simulink model "Youbot2017_2016a"  (R2022a)
settings: Solver=FixedStepAuto  StartTime=0.0  StopTime=inf  RelTol=1e-3  EnableMultiTasking=on
libraries: simulink x25, simulink_extras x7, embedlinuxNetworklib x3, dspnetwork x2
settings Model: SimulationMode=external  ExtModeTrigDuration=100  Creator=svra0001  LastModifiedBy=maximilian
settings SolverCC: AlgebraicLoopSolver=TrustRegion  PositivePriorityOrder=on  AutoInsertRateTranBlk=on
settings DataIOCC: LimitDataPoints=on  SaveFormat=Array  SignalLoggingSaveFormat=ModelDataLogs  ReturnWorkspaceOutputs=off
settings OptimizationCC: UseFloatMulNetSlope=on  EfficientFloat2IntCast=on  LifeSpan=inf  MaxStackSize=64
settings DebuggingCC: UnderspecifiedInitializationDetection=Classic  MergeDetectMultiDrivingBlocksExec=none  MultiTaskDSMMsg=warning  MultiTaskCondExecSysMsg=none  ParameterTunabilityLossMsg=error  UnconnectedInputMsg=warning  UnconnectedOutputMsg=warning  UnconnectedLineMsg=warning  AllowSymbolicDim=off  StateNameClashWarn=warning  SFUnexpectedBacktrackingDiag=warning  SFNoUnconditionalDefaultTransitionDiag=warning  SFMachineParentedDataDiag=warning  ArithmeticOperatorsInVariantConditions=warning
settings HardwareCC: ProdBitPerPointer=32  ProdBitPerSizeT=32  ProdBitPerPtrDiffT=32  ProdLargestAtomicInteger=Long  ProdLargestAtomicFloat=Double  ProdWordSize=32  ProdHWDeviceType=ARM Compatible->ARM Cortex  UseEmbeddedCoderFeatures=off  UseSimulinkCoderFeatures=off
settings ModelReferenceCC: PropagateSignalLabelsOutOfModel=off
settings SFSimCC: SimUseLocalCustomCode=off  MATLABDynamicMemAlloc=off  CustomCodeGlobalsAsFunctionIO=on  DefaultCustomCodeDeterministicFunctions=All  SimTargetLang=C++
settings RTWCC: SystemTargetFile=ert.tlc  HardwareBoard=Raspberry Pi  TLCOptions="-aInlineSetEventsForThisBaseRateFcn=TLC_FALSE -aSuppressMultiTaskScheduler=TLC_FALSE  -aRateBasedStepFcn=0"  PackageName=code.zip  TemplateMakefile=ert_default_tmf  RTWVerbose=off  RTWUseLocalCustomCode=off  Toolchain=GNU GCC Embedded Linux  DLArmComputeVersion=19.05
settings CodeAppCC: ForceParamTrailComments=on  OperatorAnnotations=on  MangleLength=10  StateflowObjectComments=on  MATLABSourceComments=on
settings ERTTargetCC: MultiwordLength=2048  ERTCustomFileBanners=off  SupportContinuousTime=on  SupportNonInlinedSFcns=on  RemoveResetFunc=off  SupportVariableSizeSignals=on  ModelStepFunctionPrototypeControlCompliant=off  ExtMode=on  ExtModeMexArgs='192.168.0.4' 1 17725  ERTSrcFileBannerTemplate=codertarget_code_template.cgt  ERTHdrFileBannerTemplate=codertarget_code_template.cgt  ERTDataSrcFileTemplate=codertarget_code_template.cgt  ERTDataHdrFileTemplate=codertarget_code_template.cgt
settings ConfigComp: CovMetricSettings=dw  CovSaveCumulativeToWorkspaceVar=on  CovSaveSingleToWorkspaceVar=on  CovExternalEMLEnable=off

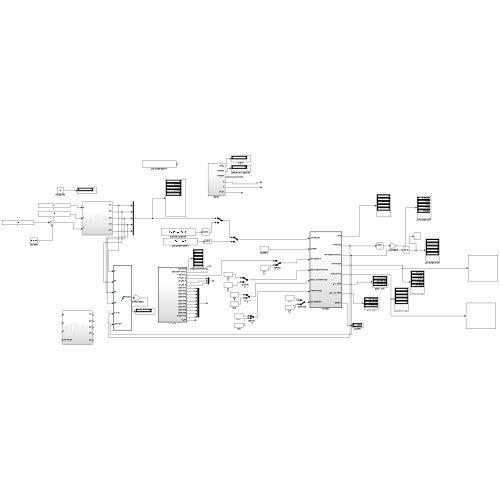
[thumbnail: Simulink's stored preview of the top-level diagram]
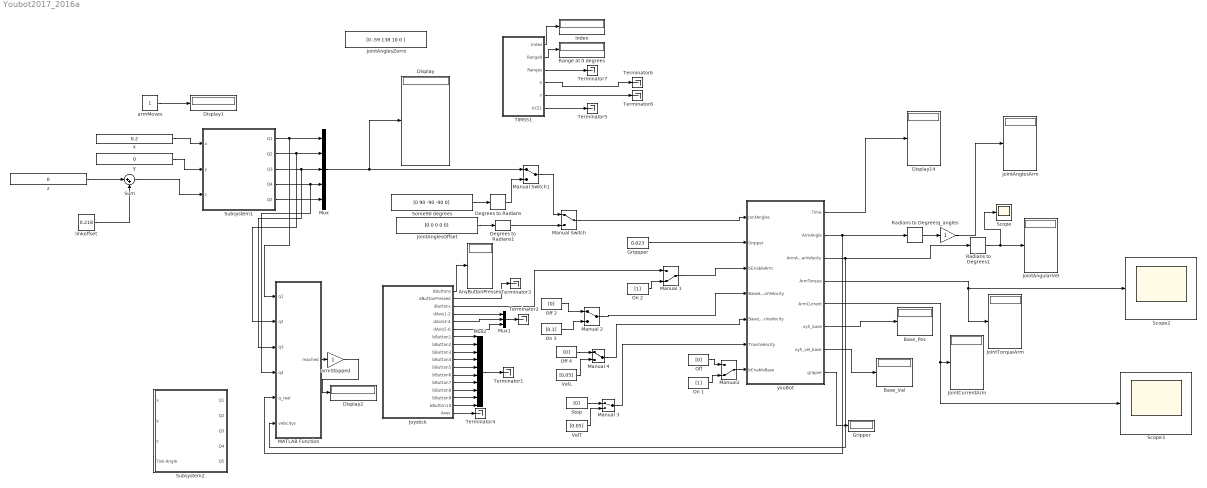
== system Youbot2017_2016a ==
  AnyButtonPressed : Display
  Base_Pos : Display
  Base_Val : Display
  Degrees to Radians : simulink_extras/Transformations/Degrees to Radians
  Degrees to Radians1 : simulink_extras/Transformations/Degrees to Radians
  Display{,1..2,14} (4 alike) : Display
  "Gripper " : Display
  Grippper : Constant  Value=0.023
  Index : Display
  JointAnglesArm : Display
  "JointAnglesOffset " : Constant  Value=[0 0 0 0 0]
  "JointAnglesZerro " : Constant  Value=[0 -59 138 10 0 ]
  JointAngularVel : Display
  JointCurrentArm : Display
  "JointTorqueArm " : Display
  "Joystick " : Subsystem  TreatAsAtomicUnit=on
      settings: RTWFcnNameOpts=Use subsystem name  RTWFileNameOpts=Use function name
  MATLAB Function : MATLAB Function  TreatAsAtomicUnit=on
  Manual 1 : ManualSwitch  CurrentSetting=0
  Manual 2 : ManualSwitch
  Manual 3 : ManualSwitch
  Manual 4 : ManualSwitch
  Manual Switch : ManualSwitch
  Manual Switch1 : ManualSwitch
  "Manual2 " : ManualSwitch  CurrentSetting=0
  Mux : Mux  Inputs=5
  Mux1 : Mux  Inputs=[2 2 2]
  Mux2 : Mux  Inputs=[1 1 1 1 1 1 1 1 1 1]
  "Off " : Constant  Value=[0]
  Off 2 : Constant  Value=[0]
  Off 4 : Constant  Value=[0]
  On 1 : Constant  Value=[1]
  On 2 : Constant  Value=[1]
  On 3 : Constant  Value=[0.1]
  Radians to Degrees : simulink_extras/Transformations/Radians to Degrees
  Radians to Degrees1 : simulink_extras/Transformations/Radians to Degrees
  "Range at 0 degrees " : Display
  Scope : Scope
  Scope2 : Scope
  Scope3 : Scope
  Some90 degrees : Constant  Value=[0 90 -90 -90 0]
  "Stop " : Constant  Value=[0]
  Subsystem1 : Subsystem
  Subsystem2 : Subsystem
  Sum : Sum  Inputs=|++
  TIM551 : Subsystem
  Terminator{1..8} (8 alike) : Terminator
  VelL : Constant  Value=[0.05]
  "VelT " : Constant  Value=[0.05]
  "armMoves " : Constant
  armStopped : Gain
  linkoffset : Constant  Value=0.218
  q_angles : Gain
  x : Constant  Value=0.2
  y : Constant  Value=0
  "youBot " : Subsystem  TreatAsAtomicUnit=on
  z : Constant  Value=0
  wires:
  Radians to Degrees/1 -> q_angles/1
  Radians to Degrees1/1 -> Scope/1, JointAngularVel/1
  "youBot "/1(Time) -> Display14/1
  "youBot "/2(ArmAngle) -> Radians to Degrees/1, MATLAB Function/5(q_real)
  "youBot "/3(ArmAngularVelocity) -> MATLAB Function/6(velocitys), Radians to Degrees1/1
  Some90 degrees/1 -> Degrees to Radians/1
  "JointAnglesOffset "/1 -> Degrees to Radians1/1
  Degrees to Radians1/1 -> Manual Switch/2
  Manual Switch/1 -> "youBot "/1(JontAngles)
  "youBot "/5(ArmCurrent) -> Scope3/1, JointCurrentArm/1
  "youBot "/4(ArmTorque) -> "JointTorqueArm "/1, Scope2/1
  "youBot "/8(gripper) -> "Gripper "/1
  "Manual2 "/1 -> "youBot "/7(bEnableBase)
  "Off "/1 -> "Manual2 "/1
  On 1/1 -> "Manual2 "/2
  On 2/1 -> Manual 1/2
  Manual 1/1 -> "youBot "/3(bEnableArm)
  Off 2/1 -> Manual 2/1
  On 3/1 -> Manual 2/2
  Manual 2/1 -> "youBot "/4("BaseAngularVelocity ")
  "Stop "/1 -> Manual 3/1
  "VelT "/1 -> Manual 3/2
  Manual 3/1 -> "youBot "/6(TransVelocity)
  Mux/1 -> Manual Switch1/1, Display/1
  Degrees to Radians/1 -> Manual Switch1/2
  Manual Switch1/1 -> Manual Switch/1
  Grippper/1 -> "youBot "/2(Gripper)
  Off 4/1 -> Manual 4/1
  VelL/1 -> Manual 4/2
  Manual 4/1 -> "youBot "/5(BaseLinearVeolocity)
  "youBot "/6(xyh_base) -> Base_Pos/1
  "youBot "/7(xyh_vel_base) -> Base_Val/1
  "Joystick "/1(bButtons) -> AnyButtonPressed/1
  "Joystick "/17(Axes) -> Terminator4/1
  "Joystick "/12(bButton6) -> Mux2/6
  "Joystick "/2("dButtonPressed ") -> Terminator3/1
  "Joystick "/7(bButton1) -> Mux2/1
  "Joystick "/8(bButton2) -> Mux2/2
  "Joystick "/9(bButton3) -> Mux2/3
  "Joystick "/10(bButton4) -> Mux2/4
  "Joystick "/11(bButton5) -> Mux2/5
  "Joystick "/13(bButton7) -> Mux2/7
  "Joystick "/14(bButton8) -> Mux2/8
  "Joystick "/15(bButton9) -> Mux2/9
  "Joystick "/16(bButton10) -> Mux2/10
  Mux2/1 -> Terminator1/1
  "Joystick "/4(dAxis1-2) -> Mux1/1
  "Joystick "/5(dAxis3-4) -> Mux1/2
  "Joystick "/6(dAxis5-6) -> Mux1/3
  Mux1/1 -> Terminator2/1
  "Joystick "/3("iButtons ") -> Manual 1/1
  TIM551/1(Index) -> Index/1
  TIM551/2(Range0) -> "Range at 0 degrees "/1
  TIM551/6(XYZ1) -> Terminator5/1
  TIM551/3(Ranges) -> Terminator7/1
  TIM551/5(Y) -> Terminator8/1
  TIM551/4(X) -> Terminator6/1
  Subsystem1/1(Q1) -> MATLAB Function/1(q1), Mux/1
  Subsystem1/3(Q3) -> MATLAB Function/3(q3), Mux/3
  Subsystem1/2(Q2) -> MATLAB Function/2(q2), Mux/2
  Subsystem1/4(Q4) -> MATLAB Function/4(q4), Mux/4
  Subsystem1/5(Q5) -> Mux/5
  "armMoves "/1 -> Display1/1
  MATLAB Function/1(reached) -> armStopped/1
  armStopped/1 -> Display2/1
  q_angles/1 -> JointAnglesArm/1
  x/1 -> Subsystem1/1(x)
  y/1 -> Subsystem1/2(y)
  z/1 -> Sum/1
  Sum/1 -> Subsystem1/3(z)
  linkoffset/1 -> Sum/2

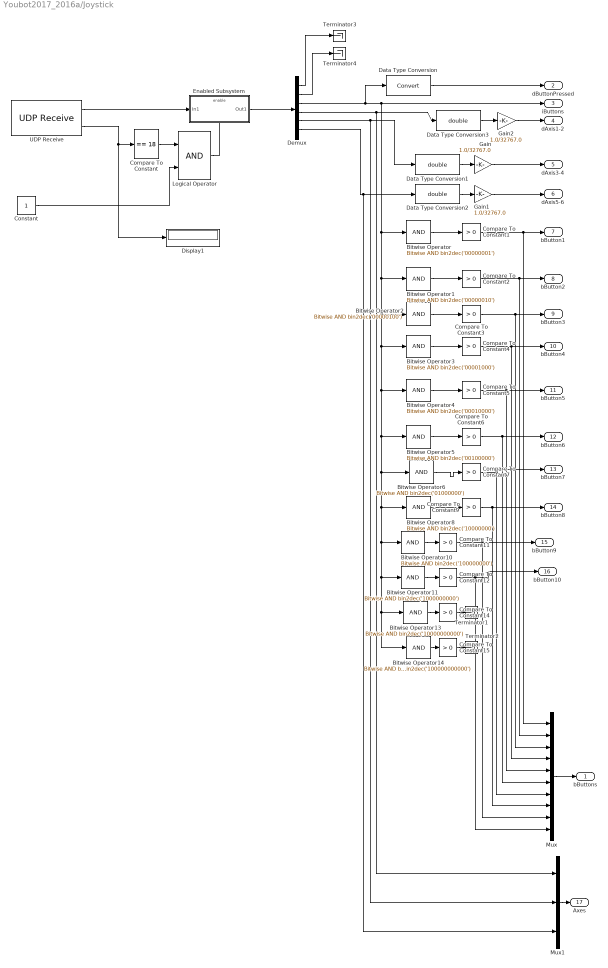
== system Youbot2017_2016a/Joystick  ==
  Bitwise Operator : simulink/Logic and Bit Operations/Bitwise Operator  logicop=AND  UseBitMask=on  BitMask=bin2dec('00000001')  BitMaskRealWorld=Stored Integer
  Bitwise Operator1 : simulink/Logic and Bit Operations/Bitwise Operator  logicop=AND  UseBitMask=on  BitMask=bin2dec('00000010')  BitMaskRealWorld=Stored Integer
  Bitwise Operator10 : simulink/Logic and Bit Operations/Bitwise Operator  logicop=AND  UseBitMask=on  BitMask=bin2dec('100000000')  BitMaskRealWorld=Stored Integer
  Bitwise Operator11 : simulink/Logic and Bit Operations/Bitwise Operator  logicop=AND  UseBitMask=on  BitMask=bin2dec('1000000000')  BitMaskRealWorld=Stored Integer
  Bitwise Operator13 : simulink/Logic and Bit Operations/Bitwise Operator  logicop=AND  UseBitMask=on  BitMask=bin2dec('10000000000')  BitMaskRealWorld=Stored Integer
  Bitwise Operator14 : simulink/Logic and Bit Operations/Bitwise Operator  logicop=AND  UseBitMask=on  BitMask=bin2dec('100000000000')  BitMaskRealWorld=Stored Integer
  Bitwise Operator2 : simulink/Logic and Bit Operations/Bitwise Operator  logicop=AND  UseBitMask=on  BitMask=bin2dec('00000100')  BitMaskRealWorld=Stored Integer
  Bitwise Operator3 : simulink/Logic and Bit Operations/Bitwise Operator  logicop=AND  UseBitMask=on  BitMask=bin2dec('00001000')  BitMaskRealWorld=Stored Integer
  Bitwise Operator4 : simulink/Logic and Bit Operations/Bitwise Operator  logicop=AND  UseBitMask=on  BitMask=bin2dec('00010000')  BitMaskRealWorld=Stored Integer
  Bitwise Operator5 : simulink/Logic and Bit Operations/Bitwise Operator  logicop=AND  UseBitMask=on  BitMask=bin2dec('00100000')  BitMaskRealWorld=Stored Integer
  Bitwise Operator6 : simulink/Logic and Bit Operations/Bitwise Operator  logicop=AND  UseBitMask=on  BitMask=bin2dec('01000000')  BitMaskRealWorld=Stored Integer
  Bitwise Operator8 : simulink/Logic and Bit Operations/Bitwise Operator  logicop=AND  UseBitMask=on  BitMask=bin2dec('10000000')  BitMaskRealWorld=Stored Integer
  Compare To Constant : simulink/Logic and Bit Operations/Compare To Constant  relop===  const=18  OutDataTypeStr=boolean
  Compare To Constant{1..7,9,11..12,14..15} (12 alike) : simulink/Logic and Bit Operations/Compare To Constant  relop=>  const=0  OutDataTypeStr=boolean
  Constant : Constant
  Data Type Conversion : DataTypeConversion  SaturateOnIntegerOverflow=off  RndMeth=Floor
  Data Type Conversion1 : DataTypeConversion  OutDataTypeStr=double  SaturateOnIntegerOverflow=off  RndMeth=Floor
  Data Type Conversion2 : DataTypeConversion  OutDataTypeStr=double  SaturateOnIntegerOverflow=off  RndMeth=Floor
  Data Type Conversion3 : DataTypeConversion  OutDataTypeStr=double  SaturateOnIntegerOverflow=off  RndMeth=Floor
  Demux : Demux  Outputs=[1 1 1 2 2 2]
  Display1 : Display
  Enabled Subsystem : Subsystem  TreatAsAtomicUnit=on
  Gain : Gain  Gain=1.0/32767.0
  Gain1 : Gain  Gain=1.0/32767.0
  Gain2 : Gain  Gain=1.0/32767.0
  Logical Operator : Logic  AllPortsSameDT=off  OutDataTypeStr=boolean
  Mux : Mux  Inputs=10
  Mux1 : Mux  Inputs=3
  Terminator{1..4} (4 alike) : Terminator
  UDP Receive : embedlinuxNetworklib/UDP Receive  localURL='0.0.0.0'  localPort=25060  remoteURL='0.0.0.0'  remotePort=-1  recvBufferSize=8192  signalDatatype=int16  dims=9  isVarSize=off  showBlockingTime=off  blockingTime=0  sampletime=0.01  blockPlatform=Raspberry Pi
      settings: SourceProductBaseCode=SC_BEAGLEBONE_BLUE,EMBEDDEDLINUX,NVIDIA,RASPPIIO
  bButtons : Outport  VectorParamsAs1DForOutWhenUnconnected=off
  "dButtonPressed " : Outport  Port=2  VectorParamsAs1DForOutWhenUnconnected=off
  "iButtons " : Outport  Port=3  VectorParamsAs1DForOutWhenUnconnected=off
  dAxis1-2 : Outport  Port=4  VectorParamsAs1DForOutWhenUnconnected=off
  dAxis3-4 : Outport  Port=5  VectorParamsAs1DForOutWhenUnconnected=off
  dAxis5-6 : Outport  Port=6  VectorParamsAs1DForOutWhenUnconnected=off
  bButton1 : Outport  Port=7  VectorParamsAs1DForOutWhenUnconnected=off
  bButton2 : Outport  Port=8  VectorParamsAs1DForOutWhenUnconnected=off
  bButton3 : Outport  Port=9  VectorParamsAs1DForOutWhenUnconnected=off
  bButton4 : Outport  Port=10  VectorParamsAs1DForOutWhenUnconnected=off
  bButton5 : Outport  Port=11  VectorParamsAs1DForOutWhenUnconnected=off
  bButton6 : Outport  Port=12  VectorParamsAs1DForOutWhenUnconnected=off
  bButton7 : Outport  Port=13  VectorParamsAs1DForOutWhenUnconnected=off
  bButton8 : Outport  Port=14  VectorParamsAs1DForOutWhenUnconnected=off
  bButton9 : Outport  Port=15  VectorParamsAs1DForOutWhenUnconnected=off
  bButton10 : Outport  Port=16  VectorParamsAs1DForOutWhenUnconnected=off
  Axes : Outport  Port=17  VectorParamsAs1DForOutWhenUnconnected=off
  wires:
  UDP Receive/2 -> Display1/1, Compare To Constant/1
  Enabled Subsystem/1(Out1) -> Demux/1
  UDP Receive/1 -> Enabled Subsystem/1(In1)
  Demux/3 -> Data Type Conversion/1, Bitwise Operator10/1, Bitwise Operator13/1, Bitwise Operator14/1, Bitwise Operator11/1, Bitwise Operator8/1, Bitwise Operator6/1, Bitwise Operator5/1, Bitwise Operator4/1, Bitwise Operator3/1, Bitwise Operator2/1, Bitwise Operator1/1, Bitwise Operator/1, "iButtons "/1
  Logical Operator/1 -> Enabled Subsystem/Enable
  Data Type Conversion/1 -> "dButtonPressed "/1
  Compare To Constant/1 -> Logical Operator/1
  Compare To Constant1/1 -> Mux/1, bButton1/1
  Bitwise Operator/1 -> Compare To Constant1/1
  Bitwise Operator5/1 -> Compare To Constant6/1
  Bitwise Operator4/1 -> Compare To Constant5/1
  Bitwise Operator3/1 -> Compare To Constant4/1
  Bitwise Operator2/1 -> Compare To Constant3/1
  Bitwise Operator1/1 -> Compare To Constant2/1
  Compare To Constant2/1 -> Mux/2, bButton2/1
  Compare To Constant3/1 -> Mux/3, bButton3/1
  Compare To Constant4/1 -> Mux/4, bButton4/1
  Compare To Constant5/1 -> Mux/5, bButton5/1
  Compare To Constant6/1 -> Mux/6, bButton6/1
  Bitwise Operator6/1 -> Compare To Constant7/1
  Compare To Constant7/1 -> Mux/7, bButton7/1
  Demux/5 -> Mux1/2, Data Type Conversion1/1
  Data Type Conversion1/1 -> Gain/1
  Gain/1 -> dAxis3-4/1
  Gain2/1 -> dAxis1-2/1
  Gain1/1 -> dAxis5-6/1
  Data Type Conversion2/1 -> Gain1/1
  Demux/6 -> Mux1/3, Data Type Conversion2/1
  Data Type Conversion3/1 -> Gain2/1
  Demux/4 -> Mux1/1, Data Type Conversion3/1
  Constant/1 -> Logical Operator/2
  Mux/1 -> bButtons/1
  Mux1/1 -> Axes/1
  Bitwise Operator8/1 -> Compare To Constant9/1
  Bitwise Operator11/1 -> Compare To Constant12/1
  Bitwise Operator14/1 -> Compare To Constant15/1
  Bitwise Operator10/1 -> Compare To Constant11/1
  Compare To Constant9/1 -> Mux/8, bButton8/1
  Compare To Constant11/1 -> Mux/9, bButton9/1
  Compare To Constant12/1 -> Mux/10, bButton10/1
  Bitwise Operator13/1 -> Compare To Constant14/1
  Compare To Constant14/1 -> Terminator1/1
  Compare To Constant15/1 -> Terminator2/1
  Demux/1 -> Terminator3/1
  Demux/2 -> Terminator4/1

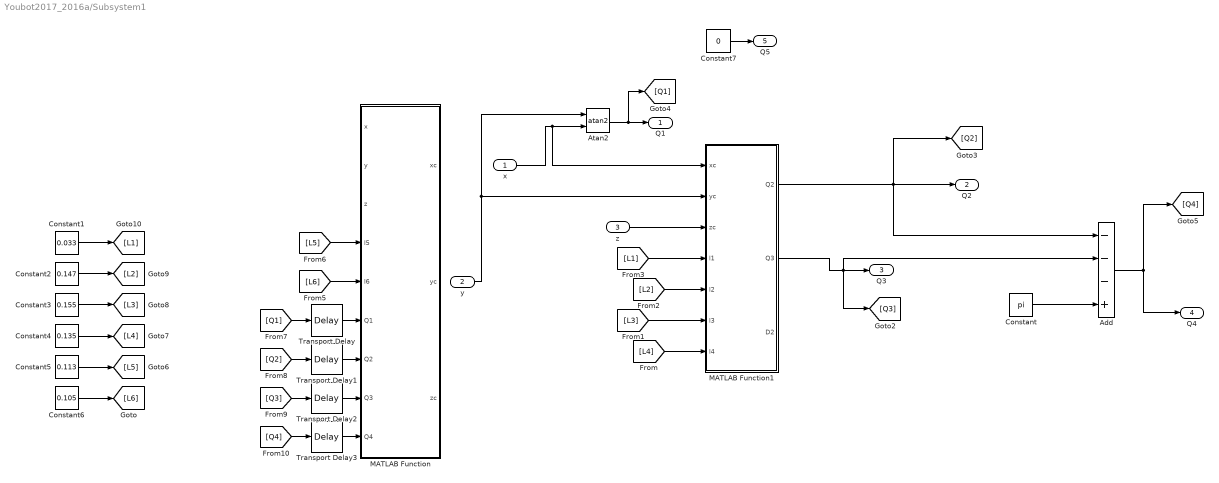
== system Youbot2017_2016a/Subsystem1 ==
  x : Inport
  y : Inport  Port=2
  z : Inport  Port=3
  Add : Sum  Inputs=---+
  Atan2 : Trigonometry  Operator=atan2
  Constant : Constant  Value=pi
  Constant1 : Constant  Value=0.033
  Constant2 : Constant  Value=0.147
  Constant3 : Constant  Value=0.155
  Constant4 : Constant  Value=0.135
  Constant5 : Constant  Value=0.113
  Constant6 : Constant  Value=0.105
  Constant7 : Constant  Value=0
  MATLAB Function : MATLAB Function  TreatAsAtomicUnit=on
  MATLAB Function1 : MATLAB Function  TreatAsAtomicUnit=on
  Transport Delay{,1..3} (4 alike) : TransportDelay
  Q1 : Outport
  Q2 : Outport  Port=2
  Q3 : Outport  Port=3
  Q4 : Outport  Port=4
  Q5 : Outport  Port=5
  wires:
  Constant2/1 -> [L2]
  [L2] -> MATLAB Function1/5(l2)
  MATLAB Function1/2(Q3) -> Add/2, Q3/1, [Q3]
  Constant/1 -> Add/4
  [L3] -> MATLAB Function1/6(l3)
  [Q1] -> Transport Delay/1
  [Q4] -> Transport Delay3/1
  Transport Delay2/1 -> MATLAB Function/8(Q3)
  Transport Delay/1 -> MATLAB Function/6(Q1)
  [L1] -> MATLAB Function1/4(l1)
  [L5] -> MATLAB Function/4(l5)
  Transport Delay1/1 -> MATLAB Function/7(Q2)
  Constant1/1 -> [L1]
  Atan2/1 -> Q1/1, [Q1]
  [Q3] -> Transport Delay2/1
  [L4] -> MATLAB Function1/7(l4)
  MATLAB Function1/1(Q2) -> Add/1, Q2/1, [Q2]
  Transport Delay3/1 -> MATLAB Function/9(Q4)
  [L6] -> MATLAB Function/5(l6)
  [Q2] -> Transport Delay1/1
  Constant4/1 -> [L4]
  Constant6/1 -> [L6]
  Constant3/1 -> [L3]
  Constant5/1 -> [L5]
  Add/1 -> Q4/1, [Q4]
  Constant7/1 -> Q5/1
  x/1 -> Atan2/2, MATLAB Function1/1(xc)
  y/1 -> MATLAB Function1/2(yc), Atan2/1
  z/1 -> MATLAB Function1/3(zc)

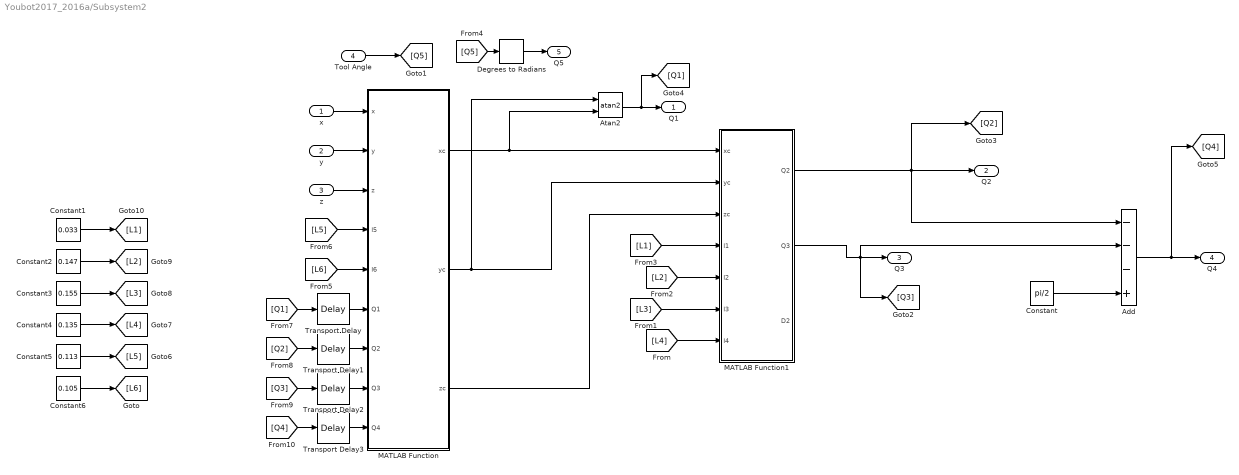
== system Youbot2017_2016a/Subsystem2 ==
  x : Inport
  y : Inport  Port=2
  z : Inport  Port=3
  Tool Angle : Inport  Port=4
  Add : Sum  Inputs=---+
  Atan2 : Trigonometry  Operator=atan2
  Constant : Constant  Value=pi/2
  Constant1 : Constant  Value=0.033
  Constant2 : Constant  Value=0.147
  Constant3 : Constant  Value=0.155
  Constant4 : Constant  Value=0.135
  Constant5 : Constant  Value=0.113
  Constant6 : Constant  Value=0.105
  Degrees to Radians : simulink_extras/Transformations/Degrees to Radians
  MATLAB Function : MATLAB Function  TreatAsAtomicUnit=on
  MATLAB Function1 : MATLAB Function  TreatAsAtomicUnit=on
  Transport Delay{,1..3} (4 alike) : TransportDelay
  Q1 : Outport
  Q2 : Outport  Port=2
  Q3 : Outport  Port=3
  Q4 : Outport  Port=4
  Q5 : Outport  Port=5
  wires:
  MATLAB Function/3(zc) -> MATLAB Function1/3(zc)
  Constant2/1 -> [L2]
  MATLAB Function/2(yc) -> Atan2/1, MATLAB Function1/2(yc)
  [L2] -> MATLAB Function1/5(l2)
  MATLAB Function1/2(Q3) -> Add/2, Q3/1, [Q3]
  Constant/1 -> Add/4
  [L3] -> MATLAB Function1/6(l3)
  [Q1] -> Transport Delay/1
  [Q4] -> Transport Delay3/1
  Transport Delay2/1 -> MATLAB Function/8(Q3)
  Transport Delay/1 -> MATLAB Function/6(Q1)
  [L1] -> MATLAB Function1/4(l1)
  [L5] -> MATLAB Function/4(l5)
  Transport Delay1/1 -> MATLAB Function/7(Q2)
  Constant1/1 -> [L1]
  Add/1 -> [Q4], Q4/1
  Atan2/1 -> Q1/1, [Q1]
  z/1 -> MATLAB Function/3(z)
  [Q3] -> Transport Delay2/1
  MATLAB Function/1(xc) -> MATLAB Function1/1(xc), Atan2/2
  x/1 -> MATLAB Function/1(x)
  [L4] -> MATLAB Function1/7(l4)
  MATLAB Function1/1(Q2) -> Add/1, Q2/1, [Q2]
  Transport Delay3/1 -> MATLAB Function/9(Q4)
  y/1 -> MATLAB Function/2(y)
  [L6] -> MATLAB Function/5(l6)
  [Q2] -> Transport Delay1/1
  Constant4/1 -> [L4]
  Constant6/1 -> [L6]
  Constant3/1 -> [L3]
  Constant5/1 -> [L5]
  Tool Angle/1 -> [Q5]
  [Q5] -> Degrees to Radians/1
  Degrees to Radians/1 -> Q5/1

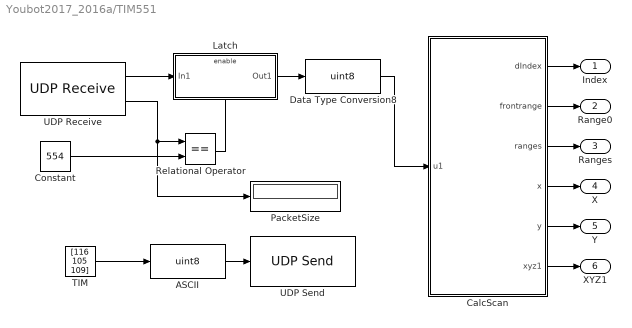
== system Youbot2017_2016a/TIM551 ==
  ASCII : DataTypeConversion  OutDataTypeStr=uint8  SaturateOnIntegerOverflow=off  RndMeth=Floor
  CalcScan : MATLAB Function  TreatAsAtomicUnit=on
  Constant : Constant  Value=554
  Data Type Conversion8 : DataTypeConversion  OutDataTypeStr=uint8  SaturateOnIntegerOverflow=off  RndMeth=Floor
  Latch : Subsystem  TreatAsAtomicUnit=on
  PacketSize : Display
  Relational Operator : RelationalOperator  Operator===  OutDataTypeStr=boolean  InputSameDT=off
  TIM : Constant  Value=[116 105 109]
  UDP Receive : dspnetwork/UDP Receive  localURL='0.0.0.0'  localPort=10000  remoteURL='0.0.0.0'  remotePort=-1  recvBufferSize=1000  dims=554  signalDatatype=int8  isComplex=off  isVarSize=off  showBlockingTime=off  blockingTime=0  sampletime=1  blockPlatform=[]
  UDP Send : dspnetwork/UDP Send  remoteURL='192.168.0.2'  remotePort=9999  localURL='0.0.0.0'  localPortSource=Automatically determine  localPort=-1  sendBufferSize=8192  sampletime=-1  blockPlatform=[]  separateLengthPort=0
  Index : Outport  VectorParamsAs1DForOutWhenUnconnected=off
  Range0 : Outport  Port=2  VectorParamsAs1DForOutWhenUnconnected=off
  Ranges : Outport  Port=3  VectorParamsAs1DForOutWhenUnconnected=off
  X : Outport  Port=4  VectorParamsAs1DForOutWhenUnconnected=off
  Y : Outport  Port=5  VectorParamsAs1DForOutWhenUnconnected=off
  XYZ1 : Outport  Port=6  VectorParamsAs1DForOutWhenUnconnected=off
  wires:
  Latch/1(Out1) -> Data Type Conversion8/1
  UDP Receive/1 -> Latch/1(In1)
  Relational Operator/1 -> Latch/Enable
  Constant/1 -> Relational Operator/2
  ASCII/1 -> UDP Send/1
  TIM/1 -> ASCII/1
  UDP Receive/2 -> PacketSize/1, Relational Operator/1
  CalcScan/2(frontrange) -> Range0/1
  Data Type Conversion8/1 -> CalcScan/1(u1)
  CalcScan/3(ranges) -> Ranges/1
  CalcScan/1(dIndex) -> Index/1
  CalcScan/6(xyz1) -> XYZ1/1
  CalcScan/5(y) -> Y/1
  CalcScan/4(x) -> X/1

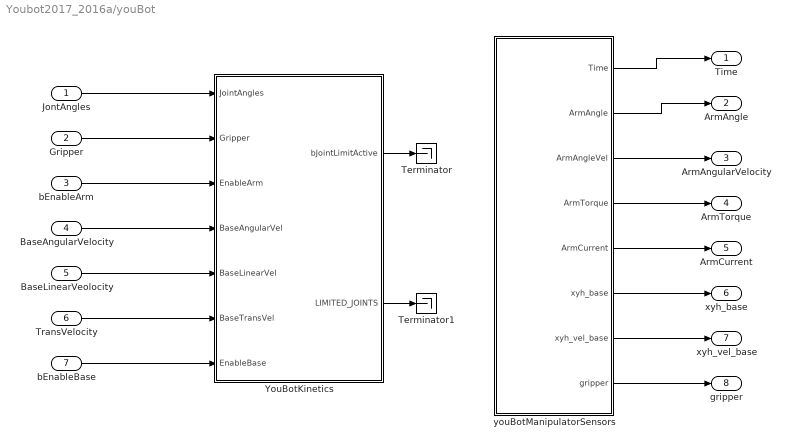
== system Youbot2017_2016a/youBot  ==
  JontAngles : Inport
  Gripper : Inport  Port=2
  bEnableArm : Inport  Port=3
  "BaseAngularVelocity " : Inport  Port=4
  BaseLinearVeolocity : Inport  Port=5
  TransVelocity : Inport  Port=6
  bEnableBase : Inport  Port=7
  Terminator : Terminator
  Terminator1 : Terminator
  "YouBotKinetics " : Subsystem
  youBotManipulatorSensors : Subsystem
  Time : Outport  VectorParamsAs1DForOutWhenUnconnected=off
  ArmAngle : Outport  Port=2  VectorParamsAs1DForOutWhenUnconnected=off
  ArmAngularVelocity : Outport  Port=3  VectorParamsAs1DForOutWhenUnconnected=off
  ArmTorque : Outport  Port=4  VectorParamsAs1DForOutWhenUnconnected=off
  ArmCurrent : Outport  Port=5  VectorParamsAs1DForOutWhenUnconnected=off
  xyh_base : Outport  Port=6  VectorParamsAs1DForOutWhenUnconnected=off
  xyh_vel_base : Outport  Port=7  VectorParamsAs1DForOutWhenUnconnected=off
  gripper : Outport  Port=8  VectorParamsAs1DForOutWhenUnconnected=off
  wires:
  JontAngles/1 -> "YouBotKinetics "/1(JointAngles)
  Gripper/1 -> "YouBotKinetics "/2(Gripper)
  bEnableArm/1 -> "YouBotKinetics "/3(EnableArm)
  "BaseAngularVelocity "/1 -> "YouBotKinetics "/4(BaseAngularVel)
  BaseLinearVeolocity/1 -> "YouBotKinetics "/5(BaseLinearVel)
  bEnableBase/1 -> "YouBotKinetics "/7("EnableBase ")
  TransVelocity/1 -> "YouBotKinetics "/6(BaseTransVel)
  youBotManipulatorSensors/1(Time) -> Time/1
  youBotManipulatorSensors/2(ArmAngle) -> ArmAngle/1
  youBotManipulatorSensors/3(ArmAngleVel) -> ArmAngularVelocity/1
  youBotManipulatorSensors/4(ArmTorque) -> ArmTorque/1
  youBotManipulatorSensors/5("ArmCurrent ") -> ArmCurrent/1
  youBotManipulatorSensors/6(xyh_base) -> xyh_base/1
  youBotManipulatorSensors/7(xyh_vel_base) -> xyh_vel_base/1
  youBotManipulatorSensors/8(gripper) -> gripper/1
  "YouBotKinetics "/1(bJointLimitActive) -> Terminator/1
  "YouBotKinetics "/2("LIMITED_JOINTS ") -> Terminator1/1

== system Youbot2017_2016a/Joystick /Enabled Subsystem ==
  In1 : Inport
  Enable : EnablePort
  Out1 : Outport  VectorParamsAs1DForOutWhenUnconnected=off
  wires:
  In1/1 -> Out1/1

== system Youbot2017_2016a/TIM551/Latch ==
  In1 : Inport
  Enable : EnablePort
  Out1 : Outport  VectorParamsAs1DForOutWhenUnconnected=off
  wires:
  In1/1 -> Out1/1

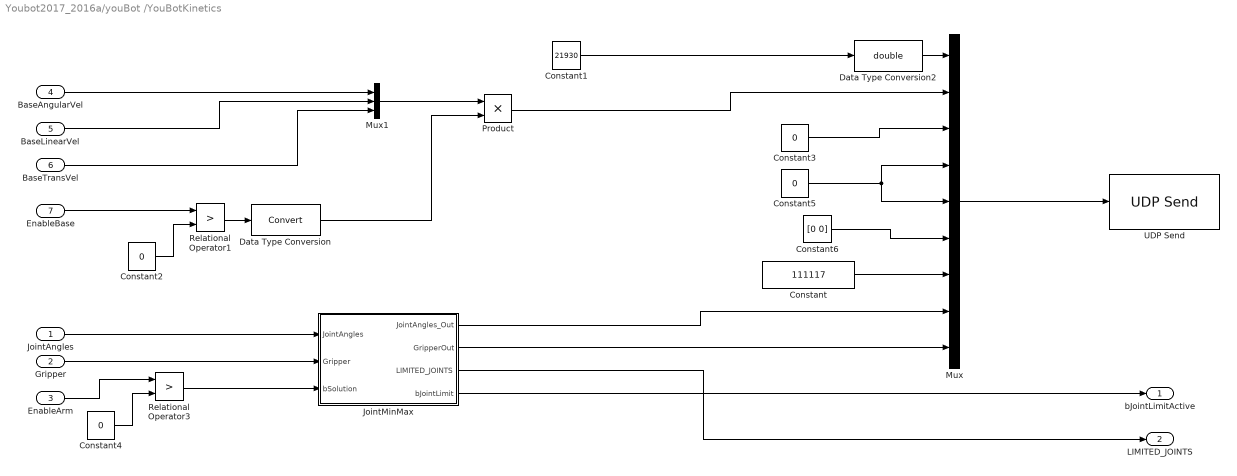
== system Youbot2017_2016a/youBot /YouBotKinetics  ==
  JointAngles : Inport
  Gripper : Inport  Port=2
  EnableArm : Inport  Port=3
  BaseAngularVel : Inport  Port=4
  BaseLinearVel : Inport  Port=5
  BaseTransVel : Inport  Port=6
  "EnableBase " : Inport  Port=7
  Constant : Constant  Value=111117
  Constant1 : Constant  Value=21930
  Constant{2..5} (4 alike) : Constant  Value=0
  Constant6 : Constant  Value=[0 0]
  Data Type Conversion : DataTypeConversion  SaturateOnIntegerOverflow=off  RndMeth=Floor
  Data Type Conversion2 : DataTypeConversion  OutDataTypeStr=double  SaturateOnIntegerOverflow=off  RndMeth=Floor
  JointMinMax : Subsystem
  Mux : Mux  Inputs=[1 3 1 1 1 2 1 5 1]
  Mux1 : Mux  Inputs=[1 1 1]
  Product : Product
  Relational Operator1 : RelationalOperator  Operator=>  OutDataTypeStr=boolean  InputSameDT=off
  Relational Operator3 : RelationalOperator  Operator=>  OutDataTypeStr=boolean  InputSameDT=off
  UDP Send : embedlinuxNetworklib/UDP Send  remoteURL='192.168.0.2'  remotePort=25005  localURL='255.255.255.255'  localPortSource=Automatically determine  localPort=-1  sampletime=-1  blockPlatform=Raspberry Pi  separateLengthPort=0
      settings: SourceProductBaseCode=SC_BEAGLEBONE_BLUE,EMBEDDEDLINUX,NVIDIA,RASPPIIO
  bJointLimitActive : Outport  VectorParamsAs1DForOutWhenUnconnected=off
  "LIMITED_JOINTS " : Outport  Port=2  VectorParamsAs1DForOutWhenUnconnected=off
  wires:
  Mux/1 -> UDP Send/1
  Data Type Conversion2/1 -> Mux/1
  Constant1/1 -> Data Type Conversion2/1
  JointMinMax/1(JointAngles_Out) -> Mux/8
  JointMinMax/2(GripperOut) -> Mux/9
  Gripper/1 -> JointMinMax/2(Gripper)
  JointAngles/1 -> JointMinMax/1(JointAngles)
  JointMinMax/3("LIMITED_JOINTS ") -> "LIMITED_JOINTS "/1
  JointMinMax/4("bJointLimit ") -> bJointLimitActive/1
  Constant/1 -> Mux/7
  BaseAngularVel/1 -> Mux1/1
  BaseLinearVel/1 -> Mux1/2
  BaseTransVel/1 -> Mux1/3
  Constant2/1 -> Relational Operator1/2
  "EnableBase "/1 -> Relational Operator1/1
  Mux1/1 -> Product/1
  Relational Operator1/1 -> Data Type Conversion/1
  Data Type Conversion/1 -> Product/2
  Product/1 -> Mux/2
  Constant4/1 -> Relational Operator3/2
  EnableArm/1 -> Relational Operator3/1
  Constant3/1 -> Mux/3
  Constant5/1 -> Mux/5, Mux/4
  Constant6/1 -> Mux/6
  Relational Operator3/1 -> JointMinMax/3(bSolution)

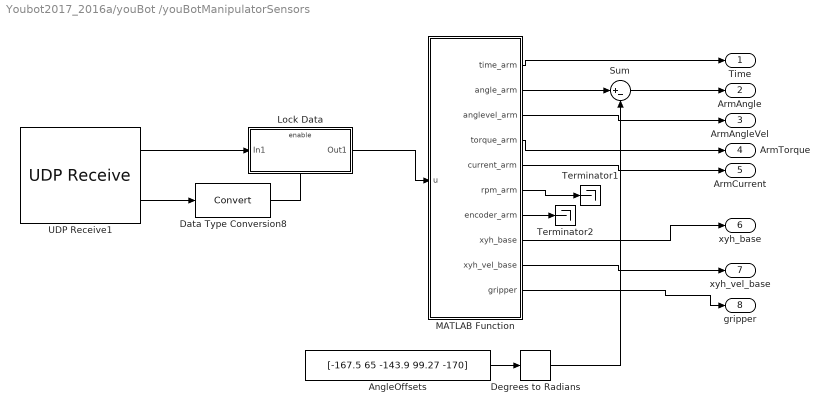
== system Youbot2017_2016a/youBot /youBotManipulatorSensors ==
  AngleOffsets : Constant  Value=[-167.5 65 -143.9 99.27 -170]
  Data Type Conversion8 : DataTypeConversion  SaturateOnIntegerOverflow=off  RndMeth=Floor
  Degrees to Radians : simulink_extras/Transformations/Degrees to Radians
  Lock Data : Subsystem  TreatAsAtomicUnit=on
  MATLAB Function : MATLAB Function  TreatAsAtomicUnit=on
  Sum : Sum  Inputs=|+-
  Terminator1 : Terminator
  Terminator2 : Terminator
  UDP Receive1 : embedlinuxNetworklib/UDP Receive  localURL='0.0.0.0'  localPort=25611  remoteURL='0.0.0.0'  remotePort=-1  recvBufferSize=8192  signalDatatype=double  dims=62  isVarSize=off  showBlockingTime=off  blockingTime=0  sampletime=0.05  blockPlatform=Raspberry Pi
      settings: SourceProductBaseCode=SC_BEAGLEBONE_BLUE,EMBEDDEDLINUX,NVIDIA,RASPPIIO
  Time : Outport  VectorParamsAs1DForOutWhenUnconnected=off
  ArmAngle : Outport  Port=2  VectorParamsAs1DForOutWhenUnconnected=off
  ArmAngleVel : Outport  Port=3  VectorParamsAs1DForOutWhenUnconnected=off
  ArmTorque : Outport  Port=4  VectorParamsAs1DForOutWhenUnconnected=off
  "ArmCurrent " : Outport  Port=5  VectorParamsAs1DForOutWhenUnconnected=off
  xyh_base : Outport  Port=6  VectorParamsAs1DForOutWhenUnconnected=off
  xyh_vel_base : Outport  Port=7  VectorParamsAs1DForOutWhenUnconnected=off
  gripper : Outport  Port=8  VectorParamsAs1DForOutWhenUnconnected=off
  wires:
  UDP Receive1/1 -> Lock Data/1(In1)
  Lock Data/1(Out1) -> MATLAB Function/1(u)
  Data Type Conversion8/1 -> Lock Data/Enable
  UDP Receive1/2 -> Data Type Conversion8/1
  MATLAB Function/1(time_arm) -> Time/1
  MATLAB Function/3(anglevel_arm) -> ArmAngleVel/1
  MATLAB Function/4(torque_arm) -> ArmTorque/1
  MATLAB Function/5(current_arm) -> "ArmCurrent "/1
  AngleOffsets/1 -> Degrees to Radians/1
  Sum/1 -> ArmAngle/1
  MATLAB Function/2(angle_arm) -> Sum/1
  Degrees to Radians/1 -> Sum/2
  MATLAB Function/8(xyh_base) -> xyh_base/1
  MATLAB Function/9(xyh_vel_base) -> xyh_vel_base/1
  MATLAB Function/10(gripper) -> gripper/1
  MATLAB Function/6(rpm_arm) -> Terminator1/1
  MATLAB Function/7(encoder_arm) -> Terminator2/1

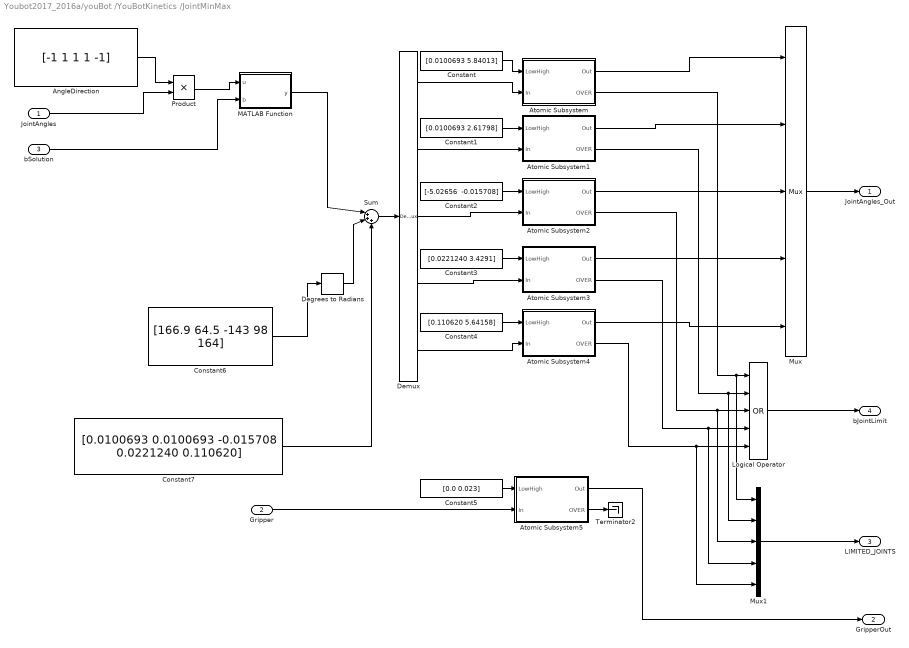
== system Youbot2017_2016a/youBot /YouBotKinetics /JointMinMax ==
  JointAngles : Inport
  Gripper : Inport  Port=2
  bSolution : Inport  Port=3
  AngleDirection : Constant  Value=[-1 1 1 1 -1]
  Atomic Subsystem : Subsystem  TreatAsAtomicUnit=on
  Atomic Subsystem1 : Subsystem  TreatAsAtomicUnit=on
  Atomic Subsystem2 : Subsystem  TreatAsAtomicUnit=on
  Atomic Subsystem3 : Subsystem  TreatAsAtomicUnit=on
  Atomic Subsystem4 : Subsystem  TreatAsAtomicUnit=on
  Atomic Subsystem5 : Subsystem  TreatAsAtomicUnit=on
  Constant : Constant  Value=[0.0100693 5.84013]
  Constant1 : Constant  Value=[0.0100693 2.61798]
  Constant2 : Constant  Value="[-5.02656  -0.015708]"
  Constant3 : Constant  Value=[0.0221240 3.4291]
  Constant4 : Constant  Value=[0.110620 5.64158]
  Constant5 : Constant  Value=[0.0 0.023]
  Constant6 : Constant  Value=[166.9 64.5 -143 98 164]
  Constant7 : Constant  Value=[0.0100693 0.0100693 -0.015708 0.0221240 0.110620]
  Degrees to Radians : simulink_extras/Transformations/Degrees to Radians
  Demux : Demux  Outputs=[ 1 1 1 1 1]
  Logical Operator : Logic  Operator=OR  Inputs=5  AllPortsSameDT=off  OutDataTypeStr=boolean
  MATLAB Function : MATLAB Function  TreatAsAtomicUnit=on
  Mux : Mux  Inputs=[1 1 1 1 1]
  Mux1 : Mux  Inputs=5
  Product : Product
  Sum : Sum  Inputs=|+++
  Terminator2 : Terminator
  JointAngles_Out : Outport  VectorParamsAs1DForOutWhenUnconnected=off
  GripperOut : Outport  Port=2  VectorParamsAs1DForOutWhenUnconnected=off
  "LIMITED_JOINTS " : Outport  Port=3  VectorParamsAs1DForOutWhenUnconnected=off
  "bJointLimit " : Outport  Port=4  VectorParamsAs1DForOutWhenUnconnected=off
  wires:
  Mux/1 -> JointAngles_Out/1
  Constant/1 -> Atomic Subsystem/1(LowHigh)
  Demux/1 -> Atomic Subsystem/2(In)
  Constant4/1 -> Atomic Subsystem4/1(LowHigh)
  Constant3/1 -> Atomic Subsystem3/1(LowHigh)
  Constant2/1 -> Atomic Subsystem2/1(LowHigh)
  Constant1/1 -> Atomic Subsystem1/1(LowHigh)
  Demux/2 -> Atomic Subsystem1/2(In)
  Atomic Subsystem/1(Out) -> Mux/1
  Demux/4 -> Atomic Subsystem3/2(In)
  Demux/3 -> Atomic Subsystem2/2(In)
  Atomic Subsystem1/1(Out) -> Mux/2
  Atomic Subsystem2/1(Out) -> Mux/3
  Atomic Subsystem3/1(Out) -> Mux/4
  Demux/5 -> Atomic Subsystem4/2(In)
  Atomic Subsystem4/1(Out) -> Mux/5
  Atomic Subsystem/2(OVER) -> Mux1/1, Logical Operator/1
  Atomic Subsystem1/2(OVER) -> Mux1/2, Logical Operator/2
  Atomic Subsystem2/2(OVER) -> Mux1/3, Logical Operator/3
  Atomic Subsystem3/2(OVER) -> Mux1/4, Logical Operator/4
  Atomic Subsystem4/2(OVER) -> Mux1/5, Logical Operator/5
  Mux1/1 -> "LIMITED_JOINTS "/1
  Gripper/1 -> Atomic Subsystem5/2(In)
  Constant5/1 -> Atomic Subsystem5/1(LowHigh)
  Sum/1 -> Demux/1
  Degrees to Radians/1 -> Sum/2
  Constant6/1 -> Degrees to Radians/1
  Constant7/1 -> Sum/3
  JointAngles/1 -> Product/2
  Logical Operator/1 -> "bJointLimit "/1
  Atomic Subsystem5/1(Out) -> GripperOut/1
  Atomic Subsystem5/2(OVER) -> Terminator2/1
  AngleDirection/1 -> Product/1
  bSolution/1 -> MATLAB Function/2(b)
  Product/1 -> MATLAB Function/1(u)
  MATLAB Function/1(y) -> Sum/1

== system Youbot2017_2016a/youBot /youBotManipulatorSensors/Lock Data ==
  In1 : Inport
  Enable : EnablePort
  Out1 : Outport  VectorParamsAs1DForOutWhenUnconnected=off
  wires:
  In1/1 -> Out1/1

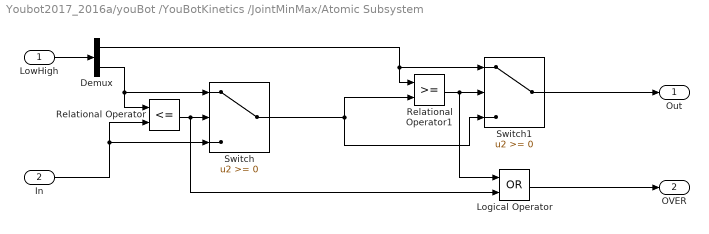
== system Youbot2017_2016a/youBot /YouBotKinetics /JointMinMax/Atomic Subsystem ==
  LowHigh : Inport
  In : Inport  Port=2
  Demux : Demux  Outputs=2
  Logical Operator : Logic  Operator=OR  AllPortsSameDT=off  OutDataTypeStr=boolean
  Relational Operator : RelationalOperator  Operator=<=  OutDataTypeStr=boolean  InputSameDT=off
  Relational Operator1 : RelationalOperator  OutDataTypeStr=boolean  InputSameDT=off
  Switch : Switch  SaturateOnIntegerOverflow=off  InputSameDT=off
  Switch1 : Switch  SaturateOnIntegerOverflow=off  InputSameDT=off
  Out : Outport  VectorParamsAs1DForOutWhenUnconnected=off
  OVER : Outport  Port=2  VectorParamsAs1DForOutWhenUnconnected=off
  wires:
  In/1 -> Relational Operator/2, Switch/3
  LowHigh/1 -> Demux/1
  Relational Operator/1 -> Logical Operator/2, Switch/2
  Demux/2 -> Switch/1, Relational Operator/1
  Switch/1 -> Switch1/3, Relational Operator1/2
  Switch1/1 -> Out/1
  Relational Operator1/1 -> Logical Operator/1, Switch1/2
  Demux/1 -> Switch1/1, Relational Operator1/1
  Logical Operator/1 -> OVER/1

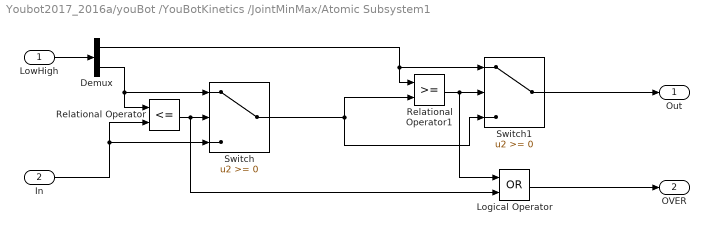
== system Youbot2017_2016a/youBot /YouBotKinetics /JointMinMax/Atomic Subsystem1 ==
  LowHigh : Inport
  In : Inport  Port=2
  Demux : Demux  Outputs=2
  Logical Operator : Logic  Operator=OR  AllPortsSameDT=off  OutDataTypeStr=boolean
  Relational Operator : RelationalOperator  Operator=<=  OutDataTypeStr=boolean  InputSameDT=off
  Relational Operator1 : RelationalOperator  OutDataTypeStr=boolean  InputSameDT=off
  Switch : Switch  SaturateOnIntegerOverflow=off  InputSameDT=off
  Switch1 : Switch  SaturateOnIntegerOverflow=off  InputSameDT=off
  Out : Outport  VectorParamsAs1DForOutWhenUnconnected=off
  OVER : Outport  Port=2  VectorParamsAs1DForOutWhenUnconnected=off
  wires:
  In/1 -> Relational Operator/2, Switch/3
  LowHigh/1 -> Demux/1
  Relational Operator/1 -> Logical Operator/2, Switch/2
  Demux/2 -> Switch/1, Relational Operator/1
  Switch/1 -> Switch1/3, Relational Operator1/2
  Switch1/1 -> Out/1
  Relational Operator1/1 -> Logical Operator/1, Switch1/2
  Demux/1 -> Switch1/1, Relational Operator1/1
  Logical Operator/1 -> OVER/1

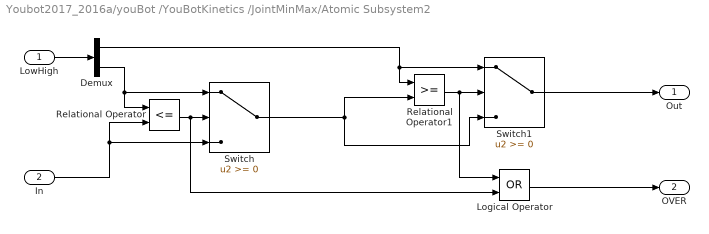
== system Youbot2017_2016a/youBot /YouBotKinetics /JointMinMax/Atomic Subsystem2 ==
  LowHigh : Inport
  In : Inport  Port=2
  Demux : Demux  Outputs=2
  Logical Operator : Logic  Operator=OR  AllPortsSameDT=off  OutDataTypeStr=boolean
  Relational Operator : RelationalOperator  Operator=<=  OutDataTypeStr=boolean  InputSameDT=off
  Relational Operator1 : RelationalOperator  OutDataTypeStr=boolean  InputSameDT=off
  Switch : Switch  SaturateOnIntegerOverflow=off  InputSameDT=off
  Switch1 : Switch  SaturateOnIntegerOverflow=off  InputSameDT=off
  Out : Outport  VectorParamsAs1DForOutWhenUnconnected=off
  OVER : Outport  Port=2  VectorParamsAs1DForOutWhenUnconnected=off
  wires:
  In/1 -> Relational Operator/2, Switch/3
  LowHigh/1 -> Demux/1
  Relational Operator/1 -> Logical Operator/2, Switch/2
  Demux/2 -> Switch/1, Relational Operator/1
  Switch/1 -> Switch1/3, Relational Operator1/2
  Switch1/1 -> Out/1
  Relational Operator1/1 -> Logical Operator/1, Switch1/2
  Demux/1 -> Switch1/1, Relational Operator1/1
  Logical Operator/1 -> OVER/1

== system Youbot2017_2016a/youBot /YouBotKinetics /JointMinMax/Atomic Subsystem3 ==
  LowHigh : Inport
  In : Inport  Port=2
  Demux : Demux  Outputs=2
  Logical Operator : Logic  Operator=OR  AllPortsSameDT=off  OutDataTypeStr=boolean
  Relational Operator : RelationalOperator  Operator=<=  OutDataTypeStr=boolean  InputSameDT=off
  Relational Operator1 : RelationalOperator  OutDataTypeStr=boolean  InputSameDT=off
  Switch : Switch  SaturateOnIntegerOverflow=off  InputSameDT=off
  Switch1 : Switch  SaturateOnIntegerOverflow=off  InputSameDT=off
  Out : Outport  VectorParamsAs1DForOutWhenUnconnected=off
  OVER : Outport  Port=2  VectorParamsAs1DForOutWhenUnconnected=off
  wires:
  In/1 -> Relational Operator/2, Switch/3
  LowHigh/1 -> Demux/1
  Relational Operator/1 -> Logical Operator/2, Switch/2
  Demux/2 -> Switch/1, Relational Operator/1
  Switch/1 -> Switch1/3, Relational Operator1/2
  Switch1/1 -> Out/1
  Relational Operator1/1 -> Logical Operator/1, Switch1/2
  Demux/1 -> Switch1/1, Relational Operator1/1
  Logical Operator/1 -> OVER/1

== system Youbot2017_2016a/youBot /YouBotKinetics /JointMinMax/Atomic Subsystem4 ==
  LowHigh : Inport
  In : Inport  Port=2
  Demux : Demux  Outputs=2
  Logical Operator : Logic  Operator=OR  AllPortsSameDT=off  OutDataTypeStr=boolean
  Relational Operator : RelationalOperator  Operator=<=  OutDataTypeStr=boolean  InputSameDT=off
  Relational Operator1 : RelationalOperator  OutDataTypeStr=boolean  InputSameDT=off
  Switch : Switch  SaturateOnIntegerOverflow=off  InputSameDT=off
  Switch1 : Switch  SaturateOnIntegerOverflow=off  InputSameDT=off
  Out : Outport  VectorParamsAs1DForOutWhenUnconnected=off
  OVER : Outport  Port=2  VectorParamsAs1DForOutWhenUnconnected=off
  wires:
  In/1 -> Relational Operator/2, Switch/3
  LowHigh/1 -> Demux/1
  Relational Operator/1 -> Logical Operator/2, Switch/2
  Demux/2 -> Switch/1, Relational Operator/1
  Switch/1 -> Switch1/3, Relational Operator1/2
  Switch1/1 -> Out/1
  Relational Operator1/1 -> Logical Operator/1, Switch1/2
  Demux/1 -> Switch1/1, Relational Operator1/1
  Logical Operator/1 -> OVER/1

== system Youbot2017_2016a/youBot /YouBotKinetics /JointMinMax/Atomic Subsystem5 ==
  LowHigh : Inport
  In : Inport  Port=2
  Demux : Demux  Outputs=2
  Logical Operator : Logic  Operator=OR  AllPortsSameDT=off  OutDataTypeStr=boolean
  Relational Operator : RelationalOperator  Operator=<=  OutDataTypeStr=boolean  InputSameDT=off
  Relational Operator1 : RelationalOperator  OutDataTypeStr=boolean  InputSameDT=off
  Switch : Switch  SaturateOnIntegerOverflow=off  InputSameDT=off
  Switch1 : Switch  SaturateOnIntegerOverflow=off  InputSameDT=off
  Out : Outport  VectorParamsAs1DForOutWhenUnconnected=off
  OVER : Outport  Port=2  VectorParamsAs1DForOutWhenUnconnected=off
  wires:
  In/1 -> Relational Operator/2, Switch/3
  LowHigh/1 -> Demux/1
  Relational Operator/1 -> Logical Operator/2, Switch/2
  Demux/2 -> Switch/1, Relational Operator/1
  Switch/1 -> Switch1/3, Relational Operator1/2
  Switch1/1 -> Out/1
  Relational Operator1/1 -> Logical Operator/1, Switch1/2
  Demux/1 -> Switch1/1, Relational Operator1/1
  Logical Operator/1 -> OVER/1

== matlab function Youbot2017_2016a/Subsystem1/MATLAB Function1 ==
  data: xc input; Q2 output; yc input; zc input; l1 input; l2 input; l3 input; l4 input; Q3 output; D2 output
function [Q2,Q3,D2] = fcn(xc,yc,zc,l1,l2,l3,l4)
D = ((xc^2+yc^2 - 2*sqrt(xc^2+yc^2)*l1 + l1^2)+(zc-l2)^2 - l3^2-l4^2)/(2*l3*l4);
D2 = 1 - D^2;
    if D2 < 0;
        Q3 = 0;
        Q2 = 0;
    else
        Q3 = atan2(sqrt(1-D^2),D);
        Q2 = atan2((sqrt(xc^2+yc^2)-l1),zc-l2) - atan2(l4*sin(Q3),l3+l4*cos(Q3));
    end

end

== matlab function Youbot2017_2016a/TIM551/CalcScan ==
  data: dIndex output; frontrange output size=1; ranges output size=271 [0..15]; x output; y output; u1 input; xyz1 output size=[4 271] [-15..15]
function [dIndex, frontrange, ranges, x, y, xyz1]  = CalcTiM551(u1)
%#codegenc
    frontrange=0;
    %ranges=zeros(1,271);
    xyz1=zeros(4,271);
    dIndex=1;
    u=zeros(271,1);
    t=u1(1:12);
    if(size(u,1)>=271)
        u=u1(13:271+12);
    end
    data=u1(1:554);
    %len=length(data);
    len=554;
    a_tim=((-135:135)*(1/270)*(pi)*(1.5))';
    index=typecast(uint8(data(1:4)),'int32')
%    timeMillis=typecast(int8(data(5:12)),'int64');
%    time=double(timeMillis)*0.001;
  %  rangesL=zeros(271,1);
  %  rangesH=zeros(271,1);
   % rangesL=double(typecast(data(13:2:len),'uint8'));
   % rangesH=double(typecast(data(14:2:len),'uint8'));
     rangesL=double(data(13:2:len));
     rangesH=double(data(14:2:len));
     %%rangesI=double(typecast([ rangesH rangesL],'uint16'));
    % ranges=ranges*0.00106;
     ranges=(rangesL+rangesH*256.0)*0.00106;
    ind=find(ranges<0.001);
    if(length(ind)>0)
        ranges(ind)=15;
    end
    
    
    num_r=length(ranges);
%     ranges=1;
%     ranges=ranges';
    x=(ranges.*cos(a_tim))';
    y=(ranges.*sin(a_tim))';
    xyz1=[x;y;zeros(1,271);ones(1,271)];
    dIndex=double(index);
    frontrange=ranges(135);
%index
%time

== matlab function Youbot2017_2016a/youBot /YouBotKinetics /JointMinMax/MATLAB Function ==
  data: u input; y output; b input
function y = fcn(u,b)
if(b>0)
    y = u;
else 
    y=0*u;
end

== matlab function Youbot2017_2016a/youBot /youBotManipulatorSensors/MATLAB Function ==
  data: u input; time_arm output; angle_arm output; anglevel_arm output; torque_arm output; current_arm output; rpm_arm output; encoder_arm output; xyh_base output; xyh_vel_base output; gripper output
function [time_arm,angle_arm, anglevel_arm, torque_arm, current_arm, rpm_arm, encoder_arm ,xyh_base,xyh_vel_base, gripper] = decodeYouBotSensorPacket(u)
    n=(0:4)*10+1;
    time_arm=u(n);
    angle_arm=u(n+1).*[-1 1 1 1 -1]';
    current_arm=u(n+2);
    torque_arm=u(n+3);
    anglevel_arm=u(n+4).*[-1 1 1 1 -1]';
    encoder_arm=u(n+5);
    rpm_arm=u(n+6);
    xyh_base=u(52:54);
    xyh_vel_base=u(55:57);
    gripper=u(61);

== matlab function Youbot2017_2016a/Subsystem2/MATLAB Function ==
  data: x input; xc output; y input; z input; l5 input; l6 input; Q1 input; Q2 input; Q3 input; Q4 input; yc output; zc output
function [xc, yc,zc] = Findoc(x,y,z,l5,l6,Q1,Q2,Q3,Q4)
 
 r13 = cos (Q1) *sin (Q2 + Q3 + Q4);
 r23 = sin (Q1) *sin (Q2 + Q3 + Q4);
 r33 = cos (Q2 + Q3 + Q4) ;

 xc=x - (l5+l6)*r13;
 yc = y - (l5+l6)*r23;
 zc = z - (l5+l6)*r33;

end

== matlab function Youbot2017_2016a/Subsystem2/MATLAB Function1 ==
  data: xc input; Q2 output; yc input; zc input; l1 input; l2 input; l3 input; l4 input; Q3 output; D2 output
function [Q2,Q3,D2] = fcn(xc,yc,zc,l1,l2,l3,l4)
D = ((xc^2+yc^2 - 2*sqrt(xc^2+yc^2)*l1 + l1^2)+(zc-l2)^2 - l3^2-l4^2)/(2*l3*l4);
D2 = 1 - D^2;
    if D2 < 0;
        Q3 = 0;
        Q2 = 0;
    else
        Q3 = atan2(sqrt(1-D^2),D);
        Q2 = atan2((sqrt(xc^2+yc^2)-l1),zc-l2) - atan2(l4*sin(Q3),l3+l4*cos(Q3));
    end

end

== matlab function Youbot2017_2016a/MATLAB Function ==
  data: reached output; q1 input; q2 input; q3 input; q4 input; q_real input; velocitys input
function reached  = fcn(q1, q2, q3, q4, q_real, velocitys)

    q1_real = q_real(1);
    q2_real = q_real(2);
    q3_real = q_real(3);
    q4_real = q_real(4);
    angles = [[q1, q1_real];[q2, q2_real]; [q3, q3_real]; [q4, q4_real]];
    reached = false;
    for i = 1:5
        if velocitys(i) ~= 0
            reached = true;
            break;
        end
    end

    if reached == false
        for i = 1:4
            if abs(angles(i,1) - angles(i,2)) > 0.1
                reached = true;
                break;
            end
        end
    end
end

== matlab function Youbot2017_2016a/Subsystem1/MATLAB Function ==
  data: x input; xc output; y input; z input; l5 input; l6 input; Q1 input; Q2 input; Q3 input; Q4 input; yc output; zc output
function [xc, yc,zc] = Findoc(x,y,z,l5,l6,Q1,Q2,Q3,Q4)
 
 r13 = cos (Q1) *sin (Q2 + Q3 + Q4);
 r23 = sin (Q1) *sin (Q2 + Q3 + Q4);
 r33 = cos (Q2 + Q3 + Q4) ;

 xc=x - (l5+l6)*r13;
 yc = y - (l5+l6)*r23;
 zc = z - (l5+l6)*r33;

end
